simulink model "PowerConverters"  (R2024b)
settings: Solver=FixedStepAuto  StartTime=0.0  StopTime=tfinal  RelTol=1e-4  EnableMultiTasking=on
PreLoadFcn:
  | PowerConvertersInit;
InitFcn:
  | PowerConvertersInit;
values from neighbouring files (symbols this model uses):
  AmplitudeVar_Buck = 50    [PowerConvertersInit.m]
  Cfilter = 200e-6    (= 0.0002)    [PowerConvertersInit.m]
  Clink_3L = Pnom_dc_3L*H_3L*2 /Vnom_dc_3L^2    (= 0.0666666666667)    [PowerConvertersInit.m]
  Clink_stat = Pnom_stat*H_stat*2 /Vnom_dc_stat^2    (= 0.0115740740741)    [PowerConvertersInit.m]
  D_Boost = 0.8    [PowerConvertersInit.m]
  D_Buck = 0.55    [PowerConvertersInit.m]
  Fnom = 60    [PowerConvertersInit.m]
  FrequencyVar_Buck = 5    [PowerConvertersInit.m]
  Fsys_FB = 50    [PowerConvertersInit.m]
  J = 10    [PowerConvertersInit.m]
  Ki_Ireg_3L = 8    [PowerConvertersInit.m]
  Ki_Ireg_motor = 0.25    [PowerConvertersInit.m]
  Ki_Ireg_stat = 80    [PowerConvertersInit.m]
  Ki_VDCreg_3L = 275    [PowerConvertersInit.m]
  Ki_VDCreg_stat = 800    [PowerConvertersInit.m]
  Ki_wreg_motor = 50    [PowerConvertersInit.m]
  Kp_Ireg_3L = 0.2/2    (= 0.1)    [PowerConvertersInit.m]
  Kp_Ireg_motor = 0.0015    [PowerConvertersInit.m]
  Kp_Ireg_stat = 0.35    [PowerConvertersInit.m]
  Kp_VDCreg_3L = 2.5    [PowerConvertersInit.m]
  Kp_VDCreg_stat = 10    [PowerConvertersInit.m]
  Kp_wreg_motor = 15    [PowerConvertersInit.m]
  Lchoke_Boost = 1e-3    (= 0.001)    [PowerConvertersInit.m]
  Lchoke_Buck = 5e-3    (= 0.005)    [PowerConvertersInit.m]
  Lchoke_FB = 1e-3    (= 0.001)    [PowerConvertersInit.m]
  Lff_3L = Lxfo_3L    (= 0.1)    [PowerConvertersInit.m]
  Lff_stat = Lxfo_Tr_stat+0.06*2    (= 0.18)    [PowerConvertersInit.m]
  Limit_Ireg_motor = [1, 0]    [PowerConvertersInit.m]
  Limit_wreg_motor = [1000, -1000]    [PowerConvertersInit.m]
  LimitL_Ireg_3L = -1.5    [PowerConvertersInit.m]
  LimitL_Ireg_stat = -1.5    [PowerConvertersInit.m]
  LimitL_VDCreg_3L = -1.5    [PowerConvertersInit.m]
  LimitL_VDCreg_stat = -1.5    [PowerConvertersInit.m]
  LimitU_Ireg_3L = 1.5    [PowerConvertersInit.m]
  LimitU_Ireg_stat = 1.5    [PowerConvertersInit.m]
  LimitU_VDCreg_3L = 1.5    [PowerConvertersInit.m]
  LimitU_VDCreg_stat = 1.5    [PowerConvertersInit.m]
  Lm_Tr_stat = 200    [PowerConvertersInit.m]
  Lstat = 0.1*Lbase_sec    (= 0.000671434916169)    [PowerConvertersInit.m]
  Lxfo_3L = 0.10    (= 0.1)    [PowerConvertersInit.m]
  Lxfo_Tr_stat = 0.06    [PowerConvertersInit.m]
  m_FB = 0.9    [PowerConvertersInit.m]
  m_HB = 1    [PowerConvertersInit.m]
  Pnom_3L = Pnom_dc_3L    (= 1000000)    [PowerConvertersInit.m]
  Pnom_dc_3L = 1e6    (= 1000000)    [PowerConvertersInit.m]
  Pnom_stat = 2e6    (= 2000000)    [PowerConvertersInit.m]
  Psc_grid = 100e6    (= 100000000)    [PowerConvertersInit.m]
  R_DCsrc = 0.5    [PowerConvertersInit.m]
  RateLimit_Iref_motor = 20000    [PowerConvertersInit.m]
  RateLimit_Qstat = Fnom*2    (= 120)    [PowerConvertersInit.m]
  RateLimit_wref_motor = 2000    [PowerConvertersInit.m]
  Rchoke_Boost = 50e-3    (= 0.05)    [PowerConvertersInit.m]
  Rchoke_Buck = 10e-3    (= 0.01)    [PowerConvertersInit.m]
  Rchoke_FB = 50e-3    (= 0.05)    [PowerConvertersInit.m]
  Rff_3L = Rxfo_3L    (= 0.00333333333333)    [PowerConvertersInit.m]
  Rff_stat = Rxfo_Tr_stat+0.06/100*2    (= 0.0032)    [PowerConvertersInit.m]
  Rfilter = 1/(Cfilter*377)/50    (= 0.26525198939)    [PowerConvertersInit.m]
  Rload_Buck = 0.1    [PowerConvertersInit.m]
  Rm_Tr_stat = 200    [PowerConvertersInit.m]
  Rstat = Lstat*(2*pi*Fnom)/100    (= 0.00253125)    [PowerConvertersInit.m]
  Rxfo_3L = 0.10/30    (= 0.00333333333333)    [PowerConvertersInit.m]
  Rxfo_Tr_stat = 0.06/30    (= 0.002)    [PowerConvertersInit.m]
  Tload = 1000    [PowerConvertersInit.m]
  Ts_Control = 50e-6    (= 5e-05)    [PowerConvertersInit.m]
  Ts_Power = 1e-7    (= 1e-07)    [PowerConvertersInit.m]
  Ts_PWM = 1e-7    (= 1e-07)    [PowerConvertersInit.m]
  V_DCsrc = 500    [PowerConvertersInit.m]
  Vload_Buck = 500    [PowerConvertersInit.m]
  Vnom_dc_3L = 1000    [PowerConvertersInit.m]
  Vnom_dc_stat = 2400    [PowerConvertersInit.m]
  Vnom_grid = 25e3    (= 25000)    [PowerConvertersInit.m]
  Vnom_prim_3L = Vnom_grid    (= 25000)    [PowerConvertersInit.m]
  Vnom_prim_stat = Vnom_grid    (= 25000)    [PowerConvertersInit.m]
  Vnom_sec_3L = 0.5*Vnom_dc_3L/sqrt(2)*sqrt(3)*m_nom_3L    [PowerConvertersInit.m]
  Vnom_sec_stat = 1800*1.25    (= 2250)    [PowerConvertersInit.m]
  wref_Initial = w_Initial*30/pi    (= 1200)    [PowerConvertersInit.m]
undefined symbols (not defined in the file or in its folder): D1, Delta, DiscIntNeverNeededParam
libraries: spsSeriesRLCBranchLib x21, spsVoltageMeasurementLib x9, spsPWMGeneratorPulseAveragingLib x7, spsCurrentMeasurementLib x5, spsMeanLib x5, spsPWMGenerator2LevelLib x4, spsPWMGeneratorDCDCLib x4, spsabctodq0Lib x4, spsSecondOrderFilterLib x4, spsLinearTransformerLib x3, spsThreePhaseVIMeasurementLib x3, spsSeriesRLCLoadLib x2
(part 1 of 2)
settings Model: SimulationMode=accelerator  Creator=The MathWorks, Inc.  LastModifiedBy=wei13
settings SolverCC: AlgebraicLoopSolver=TrustRegion  AutoInsertRateTranBlk=on
settings DataIOCC: SaveFormat=Array  SaveOutput=off  SignalLogging=off  DSMLogging=off  ReturnWorkspaceOutputs=off
settings OptimizationCC: ReuseModelBlockBuffer=off  ExpressionDepthLimit=2147483647  ZeroExternalMemoryAtStartup=off  ZeroInternalMemoryAtStartup=off  LifeSpan=inf
settings DebuggingCC: ReadBeforeWriteMsg=DisableAll  WriteAfterWriteMsg=DisableAll  WriteAfterReadMsg=DisableAll  UnderspecifiedInitializationDetection=Classic  MergeDetectMultiDrivingBlocksExec=none  TimeAdjustmentMsg=warning  MultiTaskDSMMsg=none  SingleTaskRateTransMsg=warning  VectorMatrixConversionMsg=warning  AllowSymbolicDim=off  ModelReferenceIOMismatchMessage=warning  StateNameClashWarn=warning  StrictBusMsg=WarnOnBusTreatedAsVector  NonBusSignalsTreatedAsBus=warning  SFUnexpectedBacktrackingDiag=warning  SFNoUnconditionalDefaultTransitionDiag=warning  SFExecutionAtInitializationDiag=none  ArithmeticOperatorsInVariantConditions=warning
settings HardwareCC: ProdBitPerPointer=32  ProdBitPerSizeT=32  ProdBitPerPtrDiffT=32  ProdLargestAtomicFloat=None  ProdIntDivRoundTo=Undefined  ProdEndianess=Unspecified  ProdWordSize=32  ProdHWDeviceType=32-bit Generic
settings ModelReferenceCC: UpdateModelReferenceTargets=IfOutOfDate  EnableRefExpFcnMdlSchedulingChecks=on  PropagateSignalLabelsOutOfModel=off
settings SFSimCC: SFSimEcho=off  SimUseLocalCustomCode=off  CustomCodeUndefinedFunction=UseInterfaceOnly
settings RTWCC: RTWUseLocalCustomCode=off  TargetLang=C++  GPUComputeCapability=3.5
settings CodeAppCC: StateflowObjectComments=on
settings GRTTargetCC: TargetLangStandard=C++11 (ISO)  CodeInterfacePackaging=C++ class
settings ConfigComp: CovMetricSettings=dw  CovSaveCumulativeToWorkspaceVar=on  CovSaveSingleToWorkspaceVar=on  CovExternalEMLEnable=off  CovSFcnEnable=off
settings SimscapeCC: SimscapeNormalizeSystem=off  SimscapeNominalValues={1, 'bar'; 1, 'cm^3/s'; 1, 'bar*kg/s'; 1, 'kJ/kg'; 1, 'kW'; }

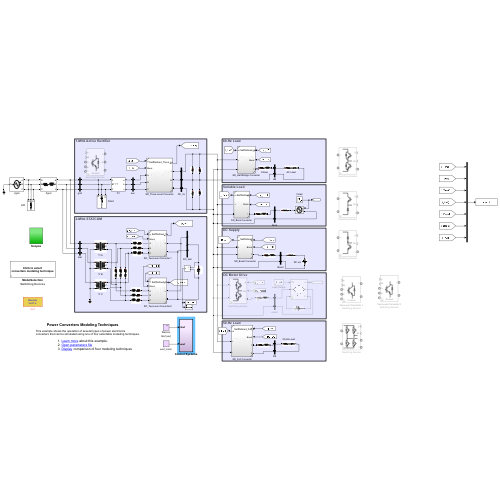
[thumbnail: Simulink's stored preview of the top-level diagram]
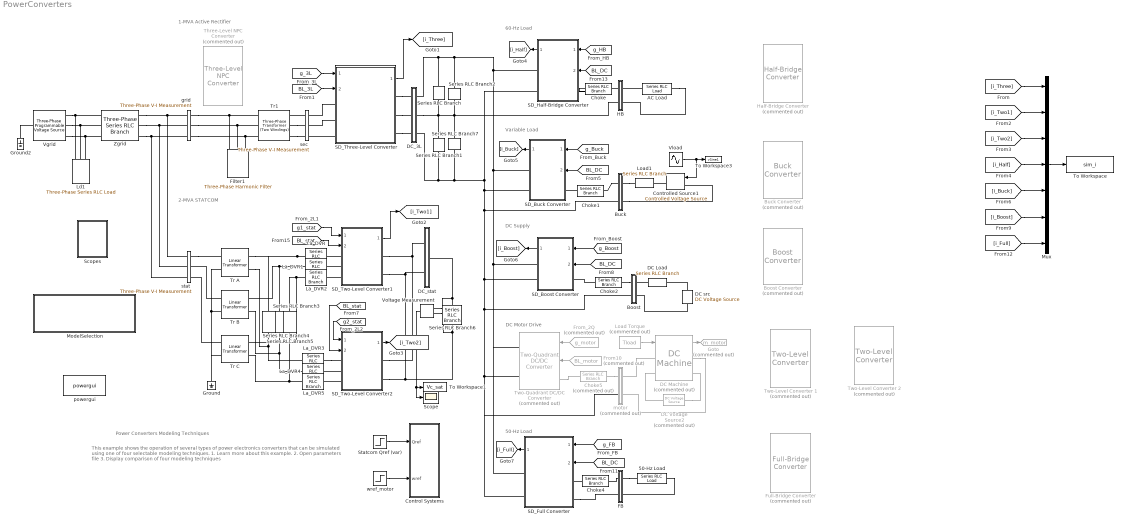
== system PowerConverters ==
  note: 50-Hz Load
  note: DC Motor Drive
  note: DC Supply
  note: 2-MVA STATCOM
  note: 1-MVA Active Rectifier
  note: Variable Load
  note: 60-Hz Load
  note: Power Converters Modeling Techniques
  note: This example shows the operation of several types of power electronics
      | converters that can be simulated using one of four selectable modeling techniques.
      |
      | 1. Learn more about this example.
      | 2. Open parameters file
      | 3. Display comparison of four modeling techniques
  50-Hz Load : spsSeriesRLCLoadLib/Series RLC Load  LConnTagsString=a  RConnTagsString=__new0  NominalVoltage=Vnom_Load_FB  NominalFrequency=Fsys_FB  ActivePower=P_Load_FB  InductivePower=0  CapacitivePower=Q_Load_FB  Setx0=off  InitialVoltage=0  SetiL0=off  InitialCurrent=0  Measurements=None  LoadType=constant Z
  AC Load : spsSeriesRLCLoadLib/Series RLC Load  LConnTagsString=a  RConnTagsString=__new0  NominalVoltage=Vnom_Load_HB  NominalFrequency=Fnom  ActivePower=P_Load_HB  InductivePower=0  CapacitivePower=Q_Load_HB  Setx0=off  InitialVoltage=0  SetiL0=off  InitialCurrent=0  Measurements=None  LoadType=constant Z
  Boost : Subsystem
  Boost Converter : spsBoostConverterLib/Boost Converter  Commented=on  ModelType=Switching devices  Ron=1e-3  Rs=1e6  Cs=inf  Vforward=[ 0, 0 ]  Ron_Diode=1e-3  Rs_Diode=1e6  Cs_Diode=inf  Vf_Diode=1e-3  Rs_CurrentSource=inf  Ron_ACsource=1e-3
      settings: AttributesFormatString=%<ModelType>
  Buck : Subsystem
  Buck Converter : spsBuckConverterLib/Buck Converter  Commented=on  ModelType=Switching devices  Ron=1e-3  Rs=1e6  Cs=inf  Vforward=[ 0, 0 ]  Ron_Diode=1e-3  Rs_Diode=1e6  Cs_Diode=inf  Vf_Diode=1e-3  Rs_CurrentSource=inf  Ron_ACsource=1e-3
      settings: AttributesFormatString=%<ModelType>
  Choke : spsSeriesRLCBranchLib/Series RLC Branch  LConnTagsString=__new0  RConnTagsString=__new0  BranchType=RL  Resistance=5e-3  Inductance=500e-6  SetiL0=off  InitialCurrent=0  Capacitance=1e-6  Setx0=off  InitialVoltage=0  Measurements=None
  Choke1 : spsSeriesRLCBranchLib/Series RLC Branch  LConnTagsString=__new0  RConnTagsString=__new0  BranchType=RL  Resistance=Rchoke_Buck  Inductance=Lchoke_Buck  SetiL0=off  InitialCurrent=0  Capacitance=1e-6  Setx0=off  InitialVoltage=0  Measurements=None
  Choke2 : spsSeriesRLCBranchLib/Series RLC Branch  LConnTagsString=__new0  RConnTagsString=__new0  BranchType=RL  Resistance=Rchoke_Boost  Inductance=Lchoke_Boost  SetiL0=off  InitialCurrent=0  Capacitance=1e-6  Setx0=off  InitialVoltage=0  Measurements=None
  Choke4 : spsSeriesRLCBranchLib/Series RLC Branch  LConnTagsString=__new0  RConnTagsString=__new0  BranchType=RL  Resistance=Rchoke_FB  Inductance=Lchoke_FB  SetiL0=off  InitialCurrent=0  Capacitance=1e-6  Setx0=off  InitialVoltage=0  Measurements=None
  Choke5 : spsSeriesRLCBranchLib/Series RLC Branch  Commented=on  LConnTagsString=__new0  RConnTagsString=__new0  BranchType=RL  Resistance=5e-3  Inductance=2e-3  SetiL0=off  InitialCurrent=0  Capacitance=1e-6  Setx0=off  InitialVoltage=0  Measurements=None
  Control Systems : Subsystem  TreatAsAtomicUnit=on  ShowSubsystemReinitializePorts=on
  Controlled Source1 : spsControlledVoltageSourceLib/Controlled Voltage Source  Initialize=on  Source_Type=AC  Amplitude=0  Phase=0  Frequency=0  Measurements=None
  DC Load : spsSeriesRLCBranchLib/Series RLC Branch  LConnTagsString=__new0  RConnTagsString=__new0  BranchType=R  Resistance=R_DCsrc  Inductance=1e-3  SetiL0=off  InitialCurrent=0  Capacitance=1e-6  Setx0=off  InitialVoltage=0  Measurements=None
  DC Machine : spsDCMachineLib/DC Machine  Commented=on  PresetModel=No  MechanicalLoad=Torque TL  FieldType=Wound  ShowDetailedParameters=on  MeasurementBus=off  RLa=Ra_La  RLf=Rf_Lf  Laf=Laf  MachineConstant=Torque constant (N.m/A)  Ke=1.8  Kt=1.8  J=J  Bm=Bm  Tf=0  w0=w_Initial  Ifinit=2.49999999368345  TsPowergui=0  TsBlock=-1
      settings: AttributesFormatString=\n
  DC Voltage Source2 : spsDCVoltageSourceLib/DC Voltage Source  Description=source block  Commented=on  Amplitude=500  Measurements=None
      settings: AttributesFormatString=\n
  DC src : spsDCVoltageSourceLib/DC Voltage Source  Amplitude=V_DCsrc  Measurements=None
  DC_3L : Subsystem
  DC_stat : Subsystem
  FB : Subsystem
  Filter1 : spsThreePhaseHarmonicFilterLib/Three-Phase Harmonic Filter  LConnTagsString=A|B|C  FilterType=Single-tuned  FilterConnection=Y (grounded)  ParNom=[Vnom_prim_3L Fnom]  Qc=Qnom_Filter1  Fr=Fn_Filter1  Frd=[11*60 13*60]  Q=Q_Filter1  Measurements=None
      settings: AttributesFormatString=\n
  From10 : From  Commented=on  GotoTag=BL_motor  TagVisibility=global
  From_2Q : From  Commented=on  GotoTag=g_motor  TagVisibility=global
  Full-Bridge Converter : spsFullBridgeConverterLib/Full-Bridge Converter  Commented=on  ModelType=Switching devices  Ron=1e-3  Rs=1e6  Cs=inf  Vforward=[ 0, 0 ]  Ron_Diode=1e-3  Rs_Diode=1e6  Cs_Diode=inf  Vf_Diode=1e-3  Rs_CurrentSource=inf  Ron_ACsource=1e-3
      settings: AttributesFormatString=%<ModelType>
  Goto : Goto  Commented=on  GotoTag=m_motor  TagVisibility=global
  Ground : spsGroundLib/Ground  LConnTagsString=a
  Ground2 : spsGroundLib/Ground  LConnTagsString=a
  HB : Subsystem
  Half-Bridge Converter : spsHalfBridgeConverterLib/Half-Bridge Converter  Commented=on  ModelType=Switching devices  Ron=1e-3  Rs=1e6  Cs=inf  Vforward=[ 0, 0 ]  Ron_Diode=1e-3  Rs_Diode=1e6  Cs_Diode=inf  Vf_Diode=1e-3  Rs_CurrentSource=inf  Ron_ACsource=1e-3
      settings: AttributesFormatString=%<ModelType>
  La_DVR{,1..5} (6 alike) : spsSeriesRLCBranchLib/Series RLC Branch  LConnTagsString=__new0  RConnTagsString=__new0  BranchType=RL  Resistance=Rstat  Inductance=Lstat  SetiL0=off  InitialCurrent=0  Capacitance=1.0  Setx0=off  InitialVoltage=0  Measurements=None
  Ld1 : spsThreePhaseSeriesRLCLoadLib/Three-Phase Series RLC Load  LConnTagsString=A|B|C  Configuration=Y (grounded)  NominalVoltage=Vnom_grid  Vabc=[1e3 1e3 1e3]  Vabcp=[1e3 1e3 1e3]  NominalFrequency=Fnom  UnbalancedPower=off  ActivePower=P_Ld1  InductivePower=0  CapacitivePower=0  Pabc=[10e3 9e3 11e3]  QLabc=[100 90 110]  QCabc=[100 90 110]  Pabcp=[10e3 9e3 11e3]  QLabcp=[100 90 110]  QCabcp=[100 90 110]  Measurements=None  LoadType=constant Z
  Load Torque : Constant  Commented=on  Value=Tload
  Load1 : spsSeriesRLCBranchLib/Series RLC Branch  LConnTagsString=__new0  RConnTagsString=__new0  BranchType=R  Resistance=Rload_Buck  Inductance=1e-3  SetiL0=off  InitialCurrent=0  Capacitance=1e-6  Setx0=off  InitialVoltage=0  Measurements=None
  ModelSelection : Subsystem  mask(Modeling Technique Selection for the power converters){SimType=Switching Devices, Ts_Control=Ts_Control, Ts_Power1=1e-7, Ts_Power2=25e-6, Ts_Power3=50e-6, Ts_PWM=25e-6}
      mask prompts: SimType "Converters modeling technique:"; Ts_Control "Control systems sample time (s)"; Ts_Power1 "SPS sample time (s):"; Ts_Power2 "SPS sample time (s):"; Ts_Power3 "SPS sample time (s):"; Ts_PWM "PWM generators sample time (s)"
      mask help:
      | We can run this example using one of the following modeling techniques:
      |
      | 1. Switching devices: The converter is modeled with IGBT/diode pairs controlled by firing pulses produced by a PWM generator.
      |
      | 2. Switching function: The converter is modeled by a switching function controlled by firing pulses produced by a PWM generator.
      |
      | 3. Switching function (PWM averaging): The converter is modeled by a switching function controlled by firing pulses produced by a PWM generator with pulse averaging. The g input then expects signals values between 0 and 1.
      |
      | 4. Average model (Uref-controlled): The converter is modeled using a switching-function model directly controlled by the reference voltage. A PWM generator is not required.
      |
      | 5. Average model (Uref-controlled, no rectifier mode): The converter is modeled using voltage sources directly controlled by the reference voltage. A PWM generator is not required, and the rectifier mode is not simulated.
      |
      | Technique 1 is the most accurate, while technique 5 yields to the fastest simulation. Technique 3 (with firing pulses averaged), as well as techniques 4 and 5 are well-suited for real-time simulation.
      mask init:
      | SystemName1=gcs;
      | PowerConvertersConfig(SystemName1, Ts_PWM, Ts_Power1, Ts_Power2, Ts_Power3, Ts_Control, SimType)
      | BlockName1=gcb;
      | switch SimType
      |     case 'Switching Devices'
      |         Color1='black';
      |     case 'Switching Function'
      |         Color1='red';
      |     case 'Switching Function (PWM averaging)'
      |         Color1='blue';
      |     case 'Average Model (Uref- or D-Controlled)'
      |         Color1='magenta';
      |     case 'Average Model (Uref- or D-Controlled, no rectifier mode)'
      |         Color1='green';
      | end
      | set_param(BlockName1,'ForegroundColor',Color1);
      | switch SimType
      |     case 1
      |         Color1='black';
      |     case 2
      |         Color1='red';
      |     case 3
      |         Color1='blue';
      |     case 4
      |         Color1='magenta';
      |     case 5
      |         Color1='green';
      | end
      | set_param(BlockName1,'ForegroundColor',Color1);
      settings: AttributesFormatString=%<SimType>
      mask TypeOptions SimType: Switching Devices | Switching Function | Switching Function (PWM averaging) | Average Model (Uref- or D-Controlled) | Average Model (Uref- or D-Controlled, no rectifier mode)
      mask Display: disp('Click to select\nconverters modeling technique')
  Mux : Mux  Inputs=7
  SD_Boost Converter : Subsystem  ReferencedSubsystem=SelfDefined_Boost_Converter
  SD_Buck Converter : Subsystem  ReferencedSubsystem=SelfDefined_Buck_Converter
  SD_Full Converter : Subsystem  ReferencedSubsystem=SelfDefined_Full_Bridge_Converter
  SD_Half-Bridge Converter : Subsystem  ReferencedSubsystem=SelfDefined_Half_Bridge_Converter
  SD_Three-Level Converter : Subsystem  ReferencedSubsystem=SelfDefined_Three_Level_NPC_Converter
  SD_Two-Level Converter1 : Subsystem  ReferencedSubsystem=SelfDefined_Two_Level_Converter
  SD_Two-Level Converter2 : Subsystem  ReferencedSubsystem=SelfDefined_Two_Level_Converter
  Scope : Scope
  Scopes : Subsystem
  Series RLC Branch : spsSeriesRLCBranchLib/Series RLC Branch  LConnTagsString=__new0  RConnTagsString=__new0  BranchType=C  Resistance=1  Inductance=1e-3  SetiL0=off  InitialCurrent=0  Capacitance=Clink_3L  Setx0=on  InitialVoltage=Vc_Initial_3L  Measurements=None
  Series RLC Branch1 : spsSeriesRLCBranchLib/Series RLC Branch  LConnTagsString=__new0  RConnTagsString=__new0  BranchType=C  Resistance=1  Inductance=1e-3  SetiL0=off  InitialCurrent=0  Capacitance=Clink_3L  Setx0=on  InitialVoltage=Vc_Initial_3L  Measurements=None
  Series RLC Branch2 : spsSeriesRLCBranchLib/Series RLC Branch  LConnTagsString=__new0  RConnTagsString=__new0  BranchType=R  Resistance=Vnom_dc_3L^2/(Pnom_dc_3L*0.01)/2  Inductance=1e-3  SetiL0=off  InitialCurrent=0  Capacitance=1e-6  Setx0=off  InitialVoltage=0  Measurements=None
  Series RLC Branch3 : spsSeriesRLCBranchLib/Series RLC Branch  LConnTagsString=__new0  RConnTagsString=__new0  BranchType=RC  Resistance=Rfilter  Inductance=1e-3  SetiL0=off  InitialCurrent=0  Capacitance=Cfilter  Setx0=off  InitialVoltage=0  Measurements=None
  Series RLC Branch4 : spsSeriesRLCBranchLib/Series RLC Branch  LConnTagsString=__new0  RConnTagsString=__new0  BranchType=RC  Resistance=Rfilter  Inductance=1e-3  SetiL0=off  InitialCurrent=0  Capacitance=Cfilter  Setx0=off  InitialVoltage=0  Measurements=None
  Series RLC Branch5 : spsSeriesRLCBranchLib/Series RLC Branch  LConnTagsString=__new0  RConnTagsString=__new0  BranchType=RC  Resistance=Rfilter  Inductance=1e-3  SetiL0=off  InitialCurrent=0  Capacitance=Cfilter  Setx0=off  InitialVoltage=0  Measurements=None
  Series RLC Branch6 : spsSeriesRLCBranchLib/Series RLC Branch  LConnTagsString=__new0  RConnTagsString=__new0  BranchType=C  Resistance=1  Inductance=1e-3  SetiL0=off  InitialCurrent=0  Capacitance=Clink_stat  Setx0=on  InitialVoltage=Vc_Initial_stat  Measurements=None
  Series RLC Branch7 : spsSeriesRLCBranchLib/Series RLC Branch  LConnTagsString=__new0  RConnTagsString=__new0  BranchType=R  Resistance=Vnom_dc_3L^2/(Pnom_dc_3L*0.01)/2  Inductance=1e-3  SetiL0=off  InitialCurrent=0  Capacitance=1e-6  Setx0=off  InitialVoltage=0  Measurements=None
  Statcom Qref (var) : Step  Time=0.6  Before=-1e6  After=1.5e6  SampleTime=Ts_Control
  Three-Level NPC Converter : spsThreeLevelNPCConverterLib/Three-Level NPC Converter  Commented=on  ModelType=Switching devices  Ron=1e-3  Rs=1e6  Cs=inf  Vforward=[ 0, 0 ]  Ron_Diode=1e-3  Rs_Diode=1e6  Cs_Diode=inf  Vf_Diode=1e-3  Rs_CurrentSource=inf  Ron_ACsource=1e-3
      settings: AttributesFormatString=%<ModelType>
  To Workspace : ToWorkspace  VariableName=sim_i  SampleTime=-1
      settings: Save2DSignal=2-D array (concatenate along first dimension)
  To Workspace1 : ToWorkspace  VariableName=Vc_sat  SampleTime=-1
      settings: Save2DSignal=2-D array (concatenate along first dimension)
  To Workspace3 : ToWorkspace  VariableName=vSine1  SampleTime=-1
      settings: Save2DSignal=2-D array (concatenate along first dimension)
  Tr A : spsLinearTransformerLib/Linear Transformer  UNITS=pu  NominalPower=[Pnom_stat/3, Fnom]  winding1="[Vnom_prim_stat/sqrt(3), Rxfo_Tr_stat/2,  Lxfo_Tr_stat/2 ]"  winding2="[Vnom_sec_stat/sqrt(3), Rxfo_Tr_stat/2,  Lxfo_Tr_stat/2 ]"  ThreeWindings=off  winding3=[60e3 0.005 0.02]  RmLm=[Rm_Tr_stat, Lm_Tr_stat]  Measurements=None  DataType=off
  Tr B : spsLinearTransformerLib/Linear Transformer  UNITS=pu  NominalPower=[Pnom_stat/3, Fnom]  winding1="[Vnom_prim_stat/sqrt(3), Rxfo_Tr_stat/2,  Lxfo_Tr_stat/2 ]"  winding2="[Vnom_sec_stat/sqrt(3), Rxfo_Tr_stat/2,  Lxfo_Tr_stat/2 ]"  ThreeWindings=off  winding3=[60e3 0.005 0.02]  RmLm=[Rm_Tr_stat, Lm_Tr_stat]  Measurements=None  DataType=off
  Tr C : spsLinearTransformerLib/Linear Transformer  UNITS=pu  NominalPower=[Pnom_stat/3, Fnom]  winding1="[Vnom_prim_stat/sqrt(3), Rxfo_Tr_stat/2,  Lxfo_Tr_stat/2 ]"  winding2="[Vnom_sec_stat/sqrt(3), Rxfo_Tr_stat/2,  Lxfo_Tr_stat/2 ]"  ThreeWindings=off  winding3=[60e3 0.005 0.02]  RmLm=[Rm_Tr_stat, Lm_Tr_stat]  Measurements=None  DataType=off
  Tr1 : spsThreePhaseTransformerTwoWindingsLib/Three-Phase Transformer (Two Windings)  Winding1Connection=Yg  Winding2Connection=Delta (D1)  CoreType=Three single-phase transformers  SetSaturation=off  Hysteresis=off  DataFile='hysteresis'  SetInitialFlux=off  Measurements=None  UNITS=pu  NominalPower="[ Pnom_3L,  Fnom ]"  Winding1=[ Vnom_prim_3L ,Rxfo_3L/2 Lxfo_3L/2 ]  Winding2=[ Vnom_sec_3L ,Rxfo_3L/2 Lxfo_3L/2 ]  Rm=Rm_3L  Lm=Lm_3L  L0=0.5  Saturation=[ 0,0 ; 0.0024,1.2 ; 1.0,1.52 ]  InitialFluxes=[ 0.8 , -0.8 , 0.7 ]  BreakLoop=off  DiscreteSolver=Trapezoidal iterative  DataType=off  TransfoNumber=1
  Two-Level Converter 1 : spsTwoLevelConverterLib/Two-Level Converter  Commented=on  ModelType=Switching devices  Ron=1e-3  Rs=1e6  Cs=inf  Vforward=[ 0, 0 ]  Ron_Diode=1e-3  Rs_Diode=1e6  Cs_Diode=inf  Vf_Diode=1e-3  Rs_CurrentSource=inf  Ron_ACsource=1e-3
      settings: AttributesFormatString=%<ModelType>
  Two-Level Converter 2 : spsTwoLevelConverterLib/Two-Level Converter  Commented=on  ModelType=Switching devices  Ron=1e-3  Rs=1e6  Cs=inf  Vforward=[ 0, 0 ]  Ron_Diode=1e-3  Rs_Diode=1e6  Cs_Diode=inf  Vf_Diode=1e-3  Rs_CurrentSource=inf  Ron_ACsource=1e-3
      settings: AttributesFormatString=%<ModelType>
  Two-Quadrant DC/DC Converter : spsTwoQuadrantDCDCConverterLib/Two-Quadrant DC//DC Converter  Commented=on  ModelType=Switching devices  Ron=1e-3  Rs=1e6  Cs=inf  Vforward=[ 0, 0 ]  Ron_Diode=1e-3  Rs_Diode=1e6  Cs_Diode=inf  Vf_Diode=1e-3  Rs_CurrentSource=inf  Ron_ACsource=1e-3
      settings: AttributesFormatString=%<ModelType>
  Vgrid : spsThreePhaseProgrammableVoltageSourceLib/Three-Phase Programmable Voltage Source  PositiveSequence=[Vnom_grid 0 Fnom]  VariationEntity=None  VariationType=Table of time-amplitude pairs  VariationTypeAlt=Step  VariationStep=0.5  VariationRate=10  VariationMagnitude=0.3  VariationFrequency=2  VariationTiming=[1 2]  VariationPhaseA=off  Amplitudes=[1 0.8 1.2 1.0]  TimeValues=[0 0.1 0.15 0.2]  HarmonicGeneration=off  HarmonicA=[1 0.05 -25 2]  HarmonicB=[1 0.0 35 2]  Timing="[0.5  0.6]"  BusType=swing  Pref=0  Qref=0  Qmin=-inf  Qmax=inf
  Vload : Sin  Amplitude=AmplitudeVar_Buck  Bias=Vload_Buck  Frequency=2*pi*FrequencyVar_Buck  SampleTime=Ts_Power
  Voltage Measurement : spsVoltageMeasurementLib/Voltage Measurement  PhasorSimulation=off  OutputType=Complex  PSBequivalent=0
  Zgrid : spsThreePhaseSeriesRLCBranchLib/Three-Phase Series RLC Branch  LConnTagsString=A|B|C  RConnTagsString=A|B|C  BranchType=RL  Resistance=Vnom_grid*Vnom_grid/Psc_grid/7  Inductance=Vnom_grid*Vnom_grid/Psc_grid/(2*pi*Fnom)  Capacitance=1e-6  Measurements=None
  grid : spsThreePhaseVIMeasurementLib/Three-Phase V-I Measurement  VoltageMeasurement=phase-to-ground  SetLabelV=on  LabelV=Vgrid  Vpu=off  VpuLL=off  CurrentMeasurement=yes  SetLabelI=on  LabelI=Igrid  Ipu=off  Pbase=100e6  Vbase=500e3  OutputType=Complex  PhasorSimulation=off  PSBequivalent=0
  motor : Subsystem  Commented=on
  powergui : spspowerguiLib/powergui  Priority=1  SimulationMode=Discrete  SampleTime=1e-7  frequency=60  Iterations=50  frequencyindice=0  Pbase=100e6  ErrMax=1e-4  UnitsV=kV  UnitsW=MW  buscounter=0  FunctionMessages=off  echomessages=off  EnableUseOfTLC=off  CurrentSourceSwitches=off  DisableSnubberDevices=off  DisableRonSwitches=off  DisableVfSwitches=off  DisplayEquations=off  AutomaticDiscreteSolvers=off  SolverType=Tustin/Backward Euler (TBE)  Interpol=off  ExternalGateDelay=off  methode=on  Ts=100  x0status=blocks  SPID=off  SwTol=0  HookPort=off  NonlinearTolerance=1e-4  nMaxIteration=100  ContinueOnMaxIteration=off  RestoreLinks=warning  ResistiveCurrentMeasurement=off  Frange=[0:2:500]  Ylog=off  Xlog=on  ShowGrid=off  save=off  variable=ZData  structure=VIPFB  ZoomFFT=on  StartTime=0.87  cycles=1  DisplayStyle=1  fundamental=50  FreqAxis=on  MaxFrequency=5000  frequencyindicesteady=1  RmsSteady=1  display=off
      settings: AttributesFormatString=%<SampleTime>
  sec : spsThreePhaseVIMeasurementLib/Three-Phase V-I Measurement  VoltageMeasurement=phase-to-phase  SetLabelV=on  LabelV=Vsec_3L_LL  Vpu=off  VpuLL=off  CurrentMeasurement=no  SetLabelI=on  LabelI=Isec  Ipu=off  Pbase=100e6  Vbase=500e3  OutputType=Complex  PhasorSimulation=off  PSBequivalent=0
  stat : spsThreePhaseVIMeasurementLib/Three-Phase V-I Measurement  VoltageMeasurement=phase-to-ground  SetLabelV=on  LabelV=Vstat  Vpu=off  VpuLL=off  CurrentMeasurement=yes  SetLabelI=on  LabelI=Istat  Ipu=off  Pbase=100e6  Vbase=500e3  OutputType=Complex  PhasorSimulation=off  PSBequivalent=0
  wref_motor : Step  Time=0.5  Before=1200  After=800  SampleTime=Ts_Control
  wires:
  From_2Q/1 -> Two-Quadrant DC/DC Converter/1
  From10/1 -> Two-Quadrant DC/DC Converter/2
  Statcom Qref (var)/1 -> Control Systems/1(Qref)
  Load Torque/1 -> DC Machine/1
  wref_motor/1 -> Control Systems/2(wref)
  DC Machine/1 -> Goto/1
  Vload/1 -> To Workspace3/1, Controlled Source1/1
  [g_3L] -> SD_Three-Level Converter/1
  [BL_3L] -> SD_Three-Level Converter/2
  [BL_stat] -> SD_Two-Level Converter1/2
  [g1_stat] -> SD_Two-Level Converter1/1
  [g2_stat] -> SD_Two-Level Converter2/1
  [BL_stat] -> SD_Two-Level Converter2/2
  [g_HB] -> SD_Half-Bridge Converter/1
  [BL_DC] -> SD_Half-Bridge Converter/2
  [BL_DC] -> SD_Buck Converter/2
  [g_Buck] -> SD_Buck Converter/1
  [BL_DC] -> SD_Boost Converter/2
  [g_Boost] -> SD_Boost Converter/1
  [g_FB] -> SD_Full Converter/1
  [BL_DC] -> SD_Full Converter/2
  SD_Three-Level Converter/1 -> [i_Three]
  SD_Two-Level Converter1/1 -> [i_Two1]
  SD_Two-Level Converter2/1 -> [i_Two2]
  SD_Half-Bridge Converter/1 -> [i_Half]
  SD_Buck Converter/1 -> [i_Buck]
  SD_Boost Converter/1 -> [i_Boost]
  SD_Full Converter/1 -> [i_Full]
  [i_Three] -> Mux/1
  [i_Two1] -> Mux/2
  [i_Two2] -> Mux/3
  [i_Half] -> Mux/4
  [i_Buck] -> Mux/5
  [i_Boost] -> Mux/6
  [i_Full] -> Mux/7
  Mux/1 -> To Workspace/1
  Voltage Measurement/1 -> To Workspace1/1, Scope/1
  connections:
  grid/LConn1 -- Filter1/LConn1 -- Tr1/LConn1
  grid/LConn2 -- Filter1/LConn2 -- Tr1/LConn2
  grid/LConn3 -- Filter1/LConn3 -- Tr1/LConn3
  sec/RConn1 -- Tr1/RConn1
  Tr1/RConn2 -- sec/RConn2
  Tr1/RConn3 -- sec/RConn3
  Vgrid/RConn2 -- Ld1/LConn2 -- Zgrid/LConn2
  Vgrid/RConn1 -- Ld1/LConn1 -- Zgrid/LConn1
  Vgrid/RConn3 -- Ld1/LConn3 -- Zgrid/LConn3
  Ground2/LConn1 -- Vgrid/LConn1
  Zgrid/RConn1 -- stat/RConn1 -- grid/RConn1
  Zgrid/RConn2 -- stat/RConn2 -- grid/RConn2
  Zgrid/RConn3 -- stat/RConn3 -- grid/RConn3
  DC_3L/RConn1 -- Series RLC Branch/LConn1 -- Series RLC Branch2/LConn1 -- SD_Half-Bridge Converter/RConn1 -- SD_Buck Converter/RConn1 -- SD_Full Converter/RConn1 -- Two-Quadrant DC/DC Converter/RConn1 -- SD_Boost Converter/RConn1
  Buck/RConn1 -- Load1/LConn1
  Two-Quadrant DC/DC Converter/LConn1 -- Choke5/LConn1
  DC src/RConn1 -- DC Load/RConn1
  Choke2/RConn1 -- Boost/LConn1
  DC Load/LConn1 -- Boost/RConn1
  DC src/LConn1 -- Boost/RConn2
  FB/RConn1 -- 50-Hz Load/LConn1
  Choke4/RConn1 -- FB/LConn1
  AC Load/LConn1 -- HB/RConn1
  AC Load/RConn1 -- HB/RConn2
  Tr A/LConn2 -- Tr B/LConn2 -- Tr C/LConn2 -- Ground/LConn1
  La_DVR/RConn1 -- Tr A/RConn1 -- Series RLC Branch4/LConn1
  SD_Two-Level Converter1/RConn1 -- SD_Two-Level Converter2/RConn1 -- DC_stat/LConn1
  Series RLC Branch6/RConn1 -- Voltage Measurement/LConn2 -- SD_Two-Level Converter1/RConn2 -- DC_stat/LConn2 -- SD_Two-Level Converter2/RConn2
  La_DVR2/RConn1 -- Series RLC Branch5/LConn1 -- Tr C/RConn1
  La_DVR1/RConn1 -- Tr B/RConn1 -- Series RLC Branch3/LConn1
  stat/LConn1 -- Tr A/LConn1
  Tr C/LConn1 -- stat/LConn3
  Tr B/LConn1 -- stat/LConn2
  Series RLC Branch6/LConn1 -- DC_stat/RConn1 -- Voltage Measurement/LConn1
  Choke/RConn1 -- HB/LConn1
  Buck/LConn2 -- Boost/LConn2 -- SD_Full Converter/RConn2 -- motor/LConn2 -- Two-Quadrant DC/DC Converter/RConn2 -- SD_Boost Converter/RConn2 -- Series RLC Branch7/RConn1 -- Series RLC Branch1/RConn1 -- DC_3L/RConn3 -- SD_Half-Bridge Converter/RConn2 -- SD_Buck Converter/RConn2
  Series RLC Branch1/LConn1 -- Series RLC Branch7/LConn1 -- HB/LConn2 -- Series RLC Branch2/RConn1 -- Series RLC Branch/RConn1 -- DC_3L/RConn2
  DC Machine/LConn1 -- motor/RConn1
  DC Voltage Source2/RConn1 -- DC Machine/LConn2
  DC Machine/RConn1 -- motor/RConn2
  DC Voltage Source2/LConn1 -- DC Machine/RConn2
  Choke5/RConn1 -- motor/LConn1
  50-Hz Load/RConn1 -- FB/RConn2
  Controlled Source1/RConn1 -- Load1/RConn1
  Series RLC Branch5/RConn1 -- Tr C/RConn2 -- La_DVR5/RConn1
  Series RLC Branch3/RConn1 -- La_DVR4/RConn1 -- Tr B/RConn2
  Series RLC Branch4/RConn1 -- Tr A/RConn2 -- La_DVR3/RConn1
  Buck/LConn1 -- Choke1/RConn1
  SD_Three-Level Converter/LConn1 -- sec/LConn1
  SD_Three-Level Converter/LConn2 -- sec/LConn2
  SD_Three-Level Converter/LConn3 -- sec/LConn3
  SD_Three-Level Converter/RConn1 -- DC_3L/LConn1
  SD_Three-Level Converter/RConn2 -- DC_3L/LConn2
  SD_Three-Level Converter/RConn3 -- DC_3L/LConn3
  SD_Two-Level Converter1/LConn1 -- La_DVR/LConn1
  SD_Two-Level Converter1/LConn2 -- La_DVR1/LConn1
  SD_Two-Level Converter1/LConn3 -- La_DVR2/LConn1
  La_DVR3/LConn1 -- SD_Two-Level Converter2/LConn1
  SD_Two-Level Converter2/LConn2 -- La_DVR4/LConn1
  SD_Two-Level Converter2/LConn3 -- La_DVR5/LConn1
  SD_Half-Bridge Converter/LConn1 -- Choke/LConn1
  Choke4/LConn1 -- SD_Full Converter/LConn1
  SD_Full Converter/LConn2 -- FB/LConn2
  Buck/RConn2 -- Controlled Source1/LConn1
  Choke1/LConn1 -- SD_Buck Converter/LConn1
  Choke2/LConn1 -- SD_Boost Converter/LConn1

== system PowerConverters/Boost ==
  CM : spsCurrentMeasurementLib/Current Measurement  PhasorSimulation=off  OutputType=Complex  PSBequivalent=0
  VM1 : spsVoltageMeasurementLib/Voltage Measurement  PhasorSimulation=off  OutputType=Complex  PSBequivalent=0
  P : PMIOPort  Side=Left
  M : PMIOPort  Port=2  Side=Left
  p : PMIOPort  Port=3  Side=Right
  m : PMIOPort  Port=4  Side=Right
  tag scope: Iboost=global, Vboost=global
  wires:
  VM1/1 -> [Vboost]
  CM/1 -> [Iboost]
  connections:
  VM1/LConn1 -- CM/LConn1 -- P/RConn1
  VM1/LConn2 -- m/RConn1 -- M/RConn1
  CM/RConn1 -- p/RConn1

== system PowerConverters/Buck ==
  CM : spsCurrentMeasurementLib/Current Measurement  PhasorSimulation=off  OutputType=Complex  PSBequivalent=0
  VM1 : spsVoltageMeasurementLib/Voltage Measurement  PhasorSimulation=off  OutputType=Complex  PSBequivalent=0
  P : PMIOPort  Side=Left
  M : PMIOPort  Port=2  Side=Left
  p : PMIOPort  Port=3  Side=Right
  m : PMIOPort  Port=4  Side=Right
  tag scope: Ibuck=global, Vbuck=global
  wires:
  CM/1 -> [Ibuck]
  VM1/1 -> [Vbuck]
  connections:
  CM/RConn1 -- p/RConn1
  m/RConn1 -- VM1/LConn2 -- M/RConn1
  CM/LConn1 -- VM1/LConn1 -- P/RConn1

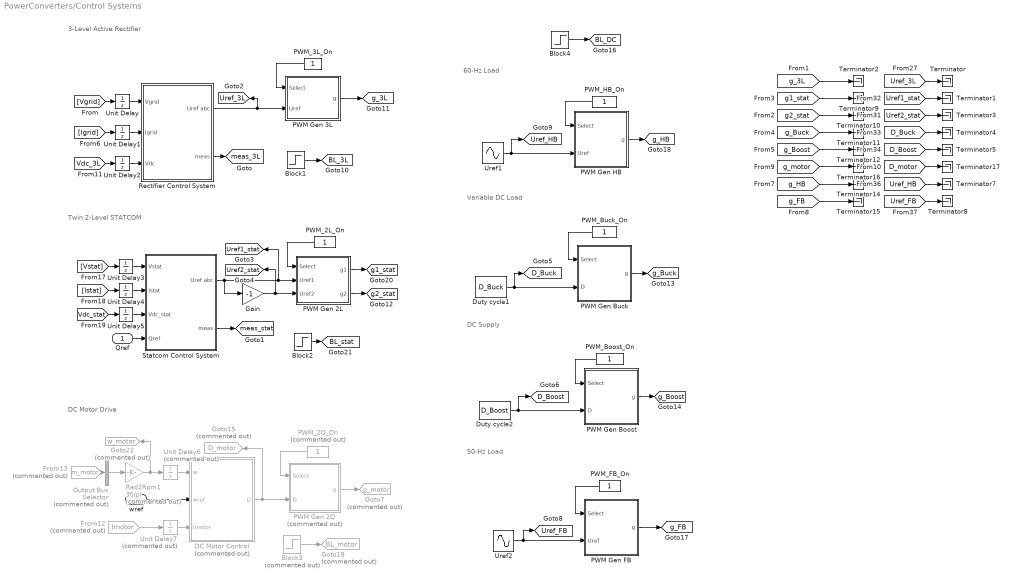
== system PowerConverters/Control Systems ==
  note: 3-Level Active Rectifier
  note: 60-Hz Load
  note: Twin 2-Level STATCOM
  note: DC Motor Drive
  note: Variable DC Load
  note: DC Supply
  note: 50-Hz Load
  Qref : Inport
  wref : Inport  Port=2
  Block1 : Step  Time=999  SampleTime=Ts_Power
  Block2 : Step  Time=999  After=0  SampleTime=Ts_Power
  Block3 : Step  Commented=on  Time=999  After=0  SampleTime=Ts_Power
  Block4 : Step  Time=0.05  Before=1  After=0  SampleTime=Ts_Power
  DC Motor Control : Subsystem  Commented=on
  Duty cycle1 : Constant  Value=D_Buck
  Duty cycle2 : Constant  Value=D_Boost
  From12 : From  Commented=on  GotoTag=Imotor  TagVisibility=global
  From13 : From  Commented=on  GotoTag=m_motor  TagVisibility=global
  Gain : Gain  Gain=-1
  Goto15 : Goto  Commented=on  GotoTag=D_motor  TagVisibility=global
  Goto19 : Goto  Commented=on  GotoTag=BL_motor  TagVisibility=global
  Goto22 : Goto  Commented=on  GotoTag=w_motor  TagVisibility=global
  Goto7 : Goto  Commented=on  GotoTag=g_motor  TagVisibility=global
  Output Bus Selector : BusSelector  Commented=on  OutputSignals=Speed wm (rad/s)  OutputAsBus=on
  PWM Gen 2L : Subsystem
  PWM Gen 2Q : Subsystem  Commented=on
  PWM Gen 3L : Subsystem
  PWM Gen Boost : Subsystem
  PWM Gen Buck : Subsystem
  PWM Gen FB : Subsystem
  PWM Gen HB : Subsystem
  PWM_2L_On : Constant
  PWM_2Q_On : Constant  Commented=on
  PWM_3L_On : Constant
      settings: AttributesFormatString=%<Tag>
  PWM_Boost_On : Constant
  PWM_Buck_On : Constant
  PWM_FB_On : Constant
  PWM_HB_On : Constant
  Rad2Rpm1 : Gain  Commented=on  Gain=30/pi  SaturateOnIntegerOverflow=on  OutDataTypeStr=Inherit: Same as input  ParamDataTypeStr=Inherit: Same as input
  Rectifier Control System : Subsystem
  Statcom Control System : Subsystem
  Terminator{,1..5,7..12,14..17} (16 alike) : Terminator
  Unit Delay{,1..5} (6 alike) : UnitDelay  SampleTime=Ts_Power  HasFrameUpgradeWarning=on
  Unit Delay6 : UnitDelay  Commented=on  SampleTime=Ts_Power  HasFrameUpgradeWarning=on
  Unit Delay7 : UnitDelay  Commented=on  SampleTime=Ts_Power  HasFrameUpgradeWarning=on
  Uref1 : Sin  Amplitude=m_HB  Frequency=2*pi*Fnom  Phase=15*pi/180  SampleTime=Ts_PWM
  Uref2 : Sin  Amplitude=m_FB  Frequency=2*pi*Fsys_FB  SampleTime=Ts_PWM
  tag scope: BL_3L=global, BL_DC=global, BL_stat=global, D_Boost=global, D_Buck=global, Uref1_stat=global, Uref2_stat=global, Uref_3L=global, Uref_FB=global, Uref_HB=global, g1_stat=global, g2_stat=global, g_3L=global, g_Boost=global, g_Buck=global, g_FB=global, g_HB=global, meas_3L=global, meas_stat=global
  wires:
  [Vdc_3L] -> Unit Delay2/1
  [Igrid] -> Unit Delay1/1
  [Vgrid] -> Unit Delay/1
  Rectifier Control System/2(meas) -> [meas_3L]
  Block1/1 -> [BL_3L]
  Block4/1 -> [BL_DC]
  Duty cycle1/1 -> [D_Buck], PWM Gen Buck/2(D)
  Duty cycle2/1 -> [D_Boost], PWM Gen Boost/2(D)
  Uref2/1 -> [Uref_FB], PWM Gen FB/2(Uref)
  Rectifier Control System/1(Uref abc) -> [Uref_3L], PWM Gen 3L/2(Uref)
  Uref1/1 -> [Uref_HB], PWM Gen HB/2(Uref)
  Gain/1 -> [Uref2_stat], PWM Gen 2L/3(Uref2)
  [Vstat] -> Unit Delay3/1
  [Vdc_stat] -> Unit Delay5/1
  Statcom Control System/2(meas) -> [meas_stat]
  [Istat] -> Unit Delay4/1
  Unit Delay/1 -> Rectifier Control System/1(Vgrid)
  Unit Delay1/1 -> Rectifier Control System/2(Igrid)
  Unit Delay2/1 -> Rectifier Control System/3(Vdc)
  Unit Delay3/1 -> Statcom Control System/1(Vstat)
  Unit Delay4/1 -> Statcom Control System/2(Istat)
  Unit Delay5/1 -> Statcom Control System/3(Vdc_stat)
  Qref/1 -> Statcom Control System/4(Qref)
  Block3/1 -> Goto19/1
  Statcom Control System/1(Uref abc) -> Gain/1, [Uref1_stat], PWM Gen 2L/2(Uref1)
  wref/1 -> DC Motor Control/2(wref)
  From12/1 -> Unit Delay7/1
  DC Motor Control/1(D) -> PWM Gen 2Q/2(D), Goto15/1
  Block2/1 -> [BL_stat]
  Unit Delay6/1 -> DC Motor Control/1(w)
  Unit Delay7/1 -> DC Motor Control/3(Imotor)
  From13/1 -> Output Bus Selector/1
  Rad2Rpm1/1 -> Goto22/1, Unit Delay6/1
  Output Bus Selector/1 -> Rad2Rpm1/1
  PWM Gen 2Q/1(g) -> Goto7/1
  PWM Gen HB/1(g) -> [g_HB]
  PWM Gen Buck/1(g) -> [g_Buck]
  PWM Gen Boost/1(g) -> [g_Boost]
  PWM Gen FB/1(g) -> [g_FB]
  PWM Gen 3L/1(g) -> [g_3L]
  PWM_3L_On/1 -> PWM Gen 3L/1(Select)
  PWM_2L_On/1 -> PWM Gen 2L/1(Select)
  PWM Gen 2L/1(g1) -> [g1_stat]
  PWM Gen 2L/2(g2) -> [g2_stat]
  PWM_2Q_On/1 -> PWM Gen 2Q/1(Select)
  PWM_HB_On/1 -> PWM Gen HB/1(Select)
  PWM_Buck_On/1 -> PWM Gen Buck/1(Select)
  PWM_Boost_On/1 -> PWM Gen Boost/1(Select)
  PWM_FB_On/1 -> PWM Gen FB/1(Select)
  [Uref_3L] -> Terminator/1
  [Uref1_stat] -> Terminator1/1
  [Uref2_stat] -> Terminator3/1
  [D_Buck] -> Terminator4/1
  [D_Boost] -> Terminator5/1
  [Uref_HB] -> Terminator7/1
  [Uref_FB] -> Terminator8/1
  [g_3L] -> Terminator2/1
  [g1_stat] -> Terminator9/1
  [g2_stat] -> Terminator10/1
  [g_Buck] -> Terminator11/1
  [g_Boost] -> Terminator12/1
  [g_HB] -> Terminator14/1
  [g_FB] -> Terminator15/1
  [g_motor] -> Terminator16/1
  [D_motor] -> Terminator17/1

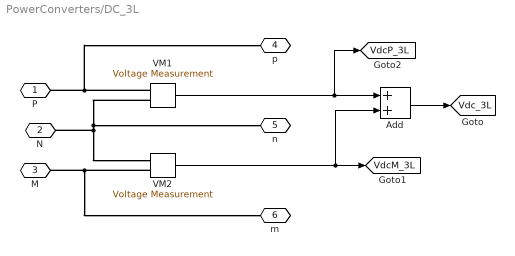
== system PowerConverters/DC_3L ==
  Add : Sum
  VM1 : spsVoltageMeasurementLib/Voltage Measurement  PhasorSimulation=off  OutputType=Complex  PSBequivalent=0
  VM2 : spsVoltageMeasurementLib/Voltage Measurement  PhasorSimulation=off  OutputType=Complex  PSBequivalent=0
  P : PMIOPort  Side=Left
  N : PMIOPort  Port=2  Side=Left
  M : PMIOPort  Port=3  Side=Left
  p : PMIOPort  Port=4  Side=Right
  n : PMIOPort  Port=5  Side=Right
  m : PMIOPort  Port=6  Side=Right
  tag scope: VdcM_3L=global, VdcP_3L=global, Vdc_3L=global
  wires:
  VM1/1 -> [VdcP_3L], Add/1
  VM2/1 -> Add/2, [VdcM_3L]
  Add/1 -> [Vdc_3L]
  connections:
  VM1/LConn1 -- p/RConn1 -- P/RConn1
  VM2/LConn2 -- m/RConn1 -- M/RConn1
  VM1/LConn2 -- VM2/LConn1 -- N/RConn1 -- n/RConn1

== system PowerConverters/DC_stat ==
  VM1 : spsVoltageMeasurementLib/Voltage Measurement  PhasorSimulation=off  OutputType=Complex  PSBequivalent=0
  P : PMIOPort  Side=Left
  M : PMIOPort  Port=2  Side=Left
  p : PMIOPort  Port=3  Side=Right
  tag scope: Vdc_stat=global
  wires:
  VM1/1 -> [Vdc_stat]
  connections:
  VM1/LConn2 -- M/RConn1
  VM1/LConn1 -- p/RConn1 -- P/RConn1

== system PowerConverters/FB ==
  CM : spsCurrentMeasurementLib/Current Measurement  PhasorSimulation=off  OutputType=Complex  PSBequivalent=0
  VM1 : spsVoltageMeasurementLib/Voltage Measurement  PhasorSimulation=off  OutputType=Complex  PSBequivalent=0
  P : PMIOPort  Side=Left
  M : PMIOPort  Port=2  Side=Left
  p : PMIOPort  Port=3  Side=Right
  m : PMIOPort  Port=4  Side=Right
  tag scope: IFB=global, VFB=global
  wires:
  CM/1 -> [IFB]
  VM1/1 -> [VFB]
  connections:
  CM/RConn1 -- p/RConn1
  M/RConn1 -- m/RConn1 -- VM1/LConn2
  P/RConn1 -- CM/LConn1 -- VM1/LConn1

== system PowerConverters/HB ==
  CM : spsCurrentMeasurementLib/Current Measurement  PhasorSimulation=off  OutputType=Complex  PSBequivalent=0
  VM1 : spsVoltageMeasurementLib/Voltage Measurement  PhasorSimulation=off  OutputType=Complex  PSBequivalent=0
  P : PMIOPort  Side=Left
  M : PMIOPort  Port=2  Side=Left
  p : PMIOPort  Port=3  Side=Right
  m : PMIOPort  Port=4  Side=Right
  tag scope: IHB=global, VHB=global
  wires:
  CM/1 -> [IHB]
  VM1/1 -> [VHB]
  connections:
  CM/RConn1 -- p/RConn1
  M/RConn1 -- m/RConn1 -- VM1/LConn2
  P/RConn1 -- CM/LConn1 -- VM1/LConn1

== system PowerConverters/ModelSelection ==

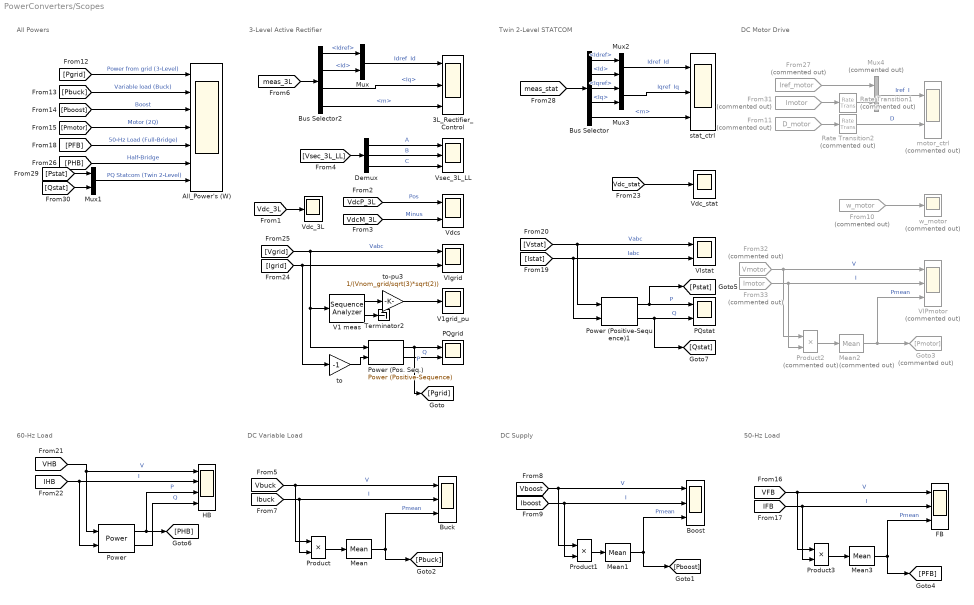
== system PowerConverters/Scopes ==
  note: DC Motor Drive
  note: Twin 2-Level STATCOM
  note: 3-Level Active Rectifier
  note: 50-Hz Load
  note: DC Supply
  note: DC Variable Load
  note: 60-Hz Load
  note: All Powers
  3L_Rectifier_Control : Scope  NumInputPorts=3
  All_Power's (W) : Scope  NumInputPorts=7
  Boost : Scope  NumInputPorts=3
  Buck : Scope  NumInputPorts=3
  Bus Selector : BusSelector  OutputSignals=Idref,Id,Iqref,Iq,m
  Bus Selector2 : BusSelector  OutputSignals=Idref,Id,Iq,m
  Demux : Demux  Outputs=3
  FB : Scope  NumInputPorts=3
  From10 : From  Commented=on  GotoTag=w_motor  TagVisibility=global
  From11 : From  Commented=on  GotoTag=D_motor  TagVisibility=global
  From27 : From  Commented=on  GotoTag=Iref_motor  TagVisibility=global
  From31 : From  Commented=on  GotoTag=Imotor  TagVisibility=global
  From32 : From  Commented=on  GotoTag=Vmotor  TagVisibility=global
  From33 : From  Commented=on  GotoTag=Imotor  TagVisibility=global
  Goto3 : Goto  Commented=on  GotoTag=Pmotor
  HB : Scope  NumInputPorts=4
  Mean : spsMeanLib/Mean  Freq=Fnom  Vinit=400e3  Ts=Ts_Power
  Mean1 : spsMeanLib/Mean  Freq=Fnom  Vinit=-100e3  Ts=Ts_Power
  Mean2 : spsMeanLib/Mean  Commented=on  Freq=Fnom  Vinit=0  Ts=Ts_Power
  Mean3 : spsMeanLib/Mean  Freq=Fsys_FB  Vinit=300e3  Ts=Ts_Power
  Mux{,1..3} (4 alike) : Mux  Inputs=2
  Mux4 : Mux  Commented=on  Inputs=2
  PQgrid : Scope  NumInputPorts=2
  PQstat : Scope  NumInputPorts=2
  Power : spsPowerLib/Power  Freq=Fnom  Vinit=[1, 0]  Iinit=[1, 0]  Ts=Ts_Power
  Power (Pos. Seq.) : spsPowerPositiveSequenceLib/Power (Positive-Sequence)  Freq=Fnom  Vinit=[Vnom_grid/sqrt(3)*sqrt(2), 0]  Iinit=[50, 0]  Ts=Ts_Power
  Power (Positive-Sequence)1 : spsPowerPositiveSequenceLib/Power (Positive-Sequence)  Freq=Fnom  Vinit=[0, 0]  Iinit=[0, 0]  Ts=Ts_Power
  Product : Product
  Product1 : Product
  Product2 : Product  Commented=on
  Product3 : Product
  Rate Transition1 : RateTransition  Commented=on  OutPortSampleTime=Ts_Control
  Rate Transition2 : RateTransition  Commented=on  OutPortSampleTime=Ts_Control
  Terminator2 : Terminator
  V1 meas : spsSequenceAnalyzerLib/Sequence Analyzer  Freq=Fnom  n=1  seq=Positive  InInit=[1, 0]  Ts=Ts_Power
  V1grid_pu : Scope
  VIPmotor : Scope  Commented=on  NumInputPorts=3
  VIgrid : Scope  NumInputPorts=2
  VIstat : Scope  NumInputPorts=2
  Vdc_3L : Scope
  Vdc_stat : Scope
  Vdcs : Scope  NumInputPorts=2
  Vsec_3L_LL : Scope  NumInputPorts=3
  motor_ctrl : Scope  Commented=on  NumInputPorts=2
  stat_ctrl : Scope  NumInputPorts=3
  to : Gain  Gain=-1
  to-pu3 : Gain  Gain=1/(Vnom_grid/sqrt(3)*sqrt(2))
  w_motor : Scope  Commented=on
  wires:
  [meas_3L] -> Bus Selector2/1
  Power (Pos. Seq.)/1 -> [Pgrid], PQgrid/1  "P"
  V1 meas/2 -> Terminator2/1
  V1 meas/1 -> to-pu3/1
  to-pu3/1 -> V1grid_pu/1
  Mux/1 -> 3L_Rectifier_Control/1  "Idref  Id"
  Bus Selector2/1 -> Mux/1  "<Idref>"
  Bus Selector2/2 -> Mux/2  "<Id>"
  Bus Selector2/4 -> 3L_Rectifier_Control/3  "<m>"
  Bus Selector2/3 -> 3L_Rectifier_Control/2  "<Iq>"
  [Vdc_3L] -> Vdc_3L/1
  [VdcP_3L] -> Vdcs/1  "Pos"
  [VdcM_3L] -> Vdcs/2  "Minus"
  [Vsec_3L_LL] -> Demux/1
  Demux/1 -> Vsec_3L_LL/1  "A"
  Demux/2 -> Vsec_3L_LL/2  "B"
  Demux/3 -> Vsec_3L_LL/3  "C"
  Power (Pos. Seq.)/2 -> PQgrid/2  "Q"
  [Vbuck] -> Product/1, Buck/1  "V"
  [Ibuck] -> Product/2, Buck/2  "I"
  Product/1 -> Mean/1
  Mean/1 -> Buck/3, [Pbuck]  "Pmean"
  [Vboost] -> Boost/1, Product1/1  "V"
  [Iboost] -> Product1/2, Boost/2  "I"
  Product1/1 -> Mean1/1
  Mean1/1 -> [Pboost], Boost/3  "Pmean"
  to/1 -> Power (Pos. Seq.)/2
  [Pgrid] -> All_Power's (W)/1  "Power from grid (3-Level)"
  [Pbuck] -> All_Power's (W)/2  "Variable load (Buck)"
  [Pboost] -> All_Power's (W)/3  "Boost"
  [Pmotor] -> All_Power's (W)/4  "Motor (2Q)"
  [VFB] -> FB/1, Product3/1  "V"
  [IFB] -> FB/2, Product3/2  "I"
  Product3/1 -> Mean3/1
  Mean3/1 -> [PFB], FB/3  "Pmean"
  [PFB] -> All_Power's (W)/5  "50-Hz Load (Full-Bridge)"
  Power (Positive-Sequence)1/1 -> [Pstat], PQstat/1  "P"
  [Vstat] -> Power (Positive-Sequence)1/1, VIstat/1  "Vabc"
  [Istat] -> Power (Positive-Sequence)1/2, VIstat/2  "Iabc"
  Power (Positive-Sequence)1/2 -> [Qstat], PQstat/2  "Q"
  [VHB] -> Power/1, HB/1  "V"
  [IHB] -> HB/2, Power/2  "I"
  Power/1 -> HB/3, [PHB]  "P"
  Power/2 -> HB/4  "Q"
  [Pstat] -> Mux1/1
  [Qstat] -> Mux1/2
  Mux1/1 -> All_Power's (W)/7  "PQ Statcom (Twin 2-Level)"
  [PHB] -> All_Power's (W)/6  "Half-Bridge"
  [Vdc_stat] -> Vdc_stat/1
  [meas_stat] -> Bus Selector/1
  Bus Selector/1 -> Mux2/1  "<Idref>"
  Bus Selector/2 -> Mux2/2  "<Id>"
  Bus Selector/3 -> Mux3/1  "<Iqref>"
  Bus Selector/4 -> Mux3/2  "<Iq>"
  Mux2/1 -> stat_ctrl/1  "Idref  Id"
  Mux3/1 -> stat_ctrl/2  "Iqref  Iq"
  Bus Selector/5 -> stat_ctrl/3  "<m>"
  From27/1 -> Mux4/1
  From31/1 -> Rate Transition1/1
  Rate Transition1/1 -> Mux4/2
  From11/1 -> Rate Transition2/1
  From32/1 -> VIPmotor/1, Product2/1  "V"
  From33/1 -> VIPmotor/2, Product2/2  "I"
  Product2/1 -> Mean2/1
  Mean2/1 -> VIPmotor/3, Goto3/1  "Pmean"
  From10/1 -> w_motor/1
  Mux4/1 -> motor_ctrl/1  "Iref  I"
  Rate Transition2/1 -> motor_ctrl/2  "D"
  [Igrid] -> VIgrid/2, to/1
  [Vgrid] -> VIgrid/1, V1 meas/1, Power (Pos. Seq.)/1  "Vabc"

== system PowerConverters/motor ==
  CM : spsCurrentMeasurementLib/Current Measurement  PhasorSimulation=off  OutputType=Complex  PSBequivalent=0
  VM1 : spsVoltageMeasurementLib/Voltage Measurement  PhasorSimulation=off  OutputType=Complex  PSBequivalent=0
  P : PMIOPort  Side=Left
  M : PMIOPort  Port=2  Side=Left
  p : PMIOPort  Port=3  Side=Right
  m : PMIOPort  Port=4  Side=Right
  tag scope: Imotor=global, Vmotor=global
  wires:
  VM1/1 -> [Vmotor]
  CM/1 -> [Imotor]
  connections:
  P/RConn1 -- VM1/LConn1 -- CM/LConn1
  M/RConn1 -- VM1/LConn2 -- m/RConn1
  CM/RConn1 -- p/RConn1

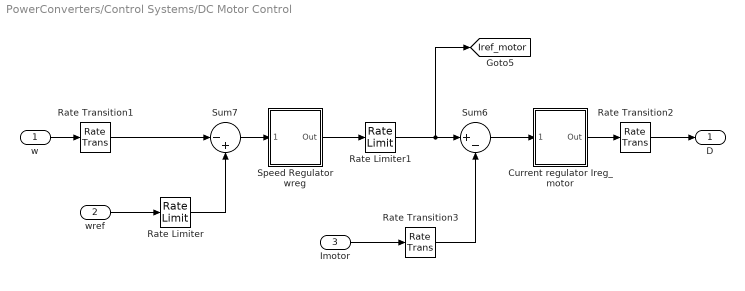
== system PowerConverters/Control Systems/DC Motor Control ==
  w : Inport
  wref : Inport  Port=2
  Imotor : Inport  Port=3
  Current regulator Ireg_motor : Subsystem  DialogController=POWERSYS.PowerSysDialog  mask(Discrete PI Controller){Kp=Kp_Ireg_motor, Ki=Ki_Ireg_motor, Par_Limits=Limit_Ireg_motor, Init=0.7, Ts=Ts_Control}
      mask prompts: Kp "Proportional gain (Kp):"; Ki "Integral gain (Ki):"; Par_Limits "Output limits: [ Upper   Lower ]"; Init "Output initial value:"; Ts "Sample time:"
      mask help: This block implements a discrete PI controller.
      mask init:
      | UpperLimit=Par_Limits(1);
      | LowerLimit=Par_Limits(2);
      | power_initmask();
      mask Help: This block is part of a subset of blocks in the Extras library that does not have documentation associated with it, other than the block mask description.
      mask Display: disp('PI');
  Rate Limiter : RateLimiter  RisingSlewLimit=RateLimit_wref_motor  FallingSlewLimit=-RateLimit_wref_motor  SampleTimeMode=inherited  InitialCondition=wref_Initial
  Rate Limiter1 : RateLimiter  RisingSlewLimit=RateLimit_Iref_motor  FallingSlewLimit=-RateLimit_Iref_motor  SampleTimeMode=inherited  InitialCondition=200
  Rate Transition1 : RateTransition  OutPortSampleTime=Ts_Control
  Rate Transition2 : RateTransition  InitialCondition=0.7  OutPortSampleTime=Ts_PWM
  Rate Transition3 : RateTransition  OutPortSampleTime=Ts_Control
  Speed Regulator wreg : Subsystem  DialogController=POWERSYS.PowerSysDialog  mask(Discrete PI Controller){Kp=Kp_wreg_motor, Ki=Ki_wreg_motor, Par_Limits=Limit_wreg_motor, Init=200, Ts=Ts_Control}
      mask prompts: Kp "Proportional gain (Kp):"; Ki "Integral gain (Ki):"; Par_Limits "Output limits: [ Upper   Lower ]"; Init "Output initial value:"; Ts "Sample time:"
      mask help: This block implements a discrete PI controller.
      mask init:
      | UpperLimit=Par_Limits(1);
      | LowerLimit=Par_Limits(2);
      | power_initmask();
      mask Help: This block is part of a subset of blocks in the Extras library that does not have documentation associated with it, other than the block mask description.
      mask Display: disp('PI');
  Sum6 : Sum  Inputs=|+-  InputSameDT=on  SaturateOnIntegerOverflow=on  OutDataTypeStr=Inherit: Same as first input
  Sum7 : Sum  Inputs=|-+  InputSameDT=on  SaturateOnIntegerOverflow=on  OutDataTypeStr=Inherit: Same as first input
  D : Outport  VectorParamsAs1DForOutWhenUnconnected=off
  tag scope: Iref_motor=global
  wires:
  w/1 -> Rate Transition1/1
  Rate Transition3/1 -> Sum6/2
  wref/1 -> Rate Limiter/1
  Sum7/1 -> Speed Regulator wreg/1(Error)
  Sum6/1 -> Current regulator Ireg_motor/1(Error)
  Rate Limiter/1 -> Sum7/2
  Speed Regulator wreg/1(Out) -> Rate Limiter1/1
  Rate Limiter1/1 -> Sum6/1, [Iref_motor]
  Imotor/1 -> Rate Transition3/1
  Current regulator Ireg_motor/1(Out) -> Rate Transition2/1
  Rate Transition1/1 -> Sum7/1
  Rate Transition2/1 -> D/1

== system PowerConverters/Control Systems/PWM Gen 2L ==
  Select : Inport
  Uref1 : Inport  Port=2
  Uref2 : Inport  Port=3
  PWMgen - Averaging : Subsystem
  Switch1 : Switch  Threshold=1.5  SaturateOnIntegerOverflow=off  InputSameDT=off
  Switch2 : Switch  Threshold=1.5  SaturateOnIntegerOverflow=off  InputSameDT=off
  g1 : Outport  VectorParamsAs1DForOutWhenUnconnected=off
  g2 : Outport  Port=2  VectorParamsAs1DForOutWhenUnconnected=off
  wires:
  Uref1/1 -> PWMgen - Averaging/1(Uref1)
  Select/1 -> Switch1/2, Switch2/2, PWMgen - Averaging/Enable
  Uref2/1 -> PWMgen - Averaging/2(Uref2)
  Switch1/1 -> g2/1
  PWMgen - Averaging/1(g1) -> Switch2/3
  PWMgen - Averaging/2(g2) -> Switch1/3
  Switch2/1 -> g1/1
  PWMgen - Averaging/3(g1_Pavg) -> Switch2/1
  PWMgen - Averaging/4(g2_Pavg) -> Switch1/1

== system PowerConverters/Control Systems/PWM Gen 2Q ==
  Select : Inport
  D : Inport  Port=2
  Subsystem : Subsystem
  Switch1 : Switch  Threshold=1.5  SaturateOnIntegerOverflow=off  InputSameDT=off
  g : Outport  VectorParamsAs1DForOutWhenUnconnected=off
  wires:
  D/1 -> Subsystem/1(D)
  Select/1 -> Switch1/2, Subsystem/Enable
  Switch1/1 -> g/1
  Subsystem/1(g) -> Switch1/3
  Subsystem/2(g_Pavg) -> Switch1/1

== system PowerConverters/Control Systems/PWM Gen 3L ==
  Select : Inport
  Uref : Inport  Port=2
  PWMgen - Averaging : Subsystem
  Switch : Switch  Threshold=1.5  SaturateOnIntegerOverflow=off  InputSameDT=off
  g : Outport  VectorParamsAs1DForOutWhenUnconnected=off
  wires:
  Select/1 -> PWMgen - Averaging/Enable, Switch/2
  Switch/1 -> g/1
  PWMgen - Averaging/2(P) -> Switch/3
  Uref/1 -> PWMgen - Averaging/1(Uref)
  PWMgen - Averaging/1(Pavg) -> Switch/1
